simulink model "pendel_2016b"  (R2016b)
settings: Solver=ode45  StartTime=0.0  StopTime=30  RelTol=1e-5  AbsTol=1e-6
values from neighbouring files (symbols this model uses):
  fmax = 10    [pendel3.mat]
  g = 9.8    [pendel3.mat]    (also in stuff.m = 9.82)
  K = acker(A, B, P)    [stuff.m]
  l = 0.7    [pendel3.mat]    (also in stuff.m)
  L_1 = -10/(pi/6)    (= -19.098593171)    [stuff.m]
  L_2 = -8    [stuff.m]
  lam1 = -0.255    [pendel3.mat]
  m = 0.05    [pendel3.mat]
  M = 0.5    [pendel3.mat]    (also in stuff.m)
  ws = 1    [pendel3.mat]
  zs = 0.7    [pendel3.mat]
libraries: simulink x1
settings Model: ExtModeTrigMode=oneshot  ExtModeArmWhenConnect=off  Creator=bruze  LastModifiedBy=viktor
settings DataIOCC: SaveFormat=Array  SignalLoggingSaveFormat=ModelDataLogs
settings OptimizationCC: BlockReduction=off  BooleanDataType=off  ExpressionDepthLimit=2147483647  LifeSpan=inf
settings DebuggingCC: SaveWithParameterizedLinksMsg=none  UnderspecifiedInitializationDetection=Classic  MergeDetectMultiDrivingBlocksExec=none  SignalResolutionControl=TryResolveAllWithWarning  MultiTaskDSMMsg=warning  MultiTaskCondExecSysMsg=none  StateNameClashWarn=warning  SFUnexpectedBacktrackingDiag=warning  SFNoUnconditionalDefaultTransitionDiag=warning  SFExecutionAtInitializationDiag=none
settings HardwareCC: ProdBitPerPointer=32  ProdBitPerSizeT=32  ProdBitPerPtrDiffT=32  ProdLargestAtomicFloat=None  ProdIntDivRoundTo=Undefined  ProdEndianess=Unspecified  ProdWordSize=32  ProdHWDeviceType=32-bit Generic  TargetUnknown=on
settings ModelReferenceCC: PropagateSignalLabelsOutOfModel=off
settings GRTTargetCC: TargetLangStandard=C89/C90 (ANSI)  GeneratePreprocessorConditionals=Disable all  CombineOutputUpdateFcns=off  GRTInterface=on
settings ConfigComp: CovMetricSettings=dw  CovHtmlReporting=on  CovSaveCumulativeToWorkspaceVar=on  CovSaveSingleToWorkspaceVar=on  CovExternalEMLEnable=off  CovSFcnEnable=off

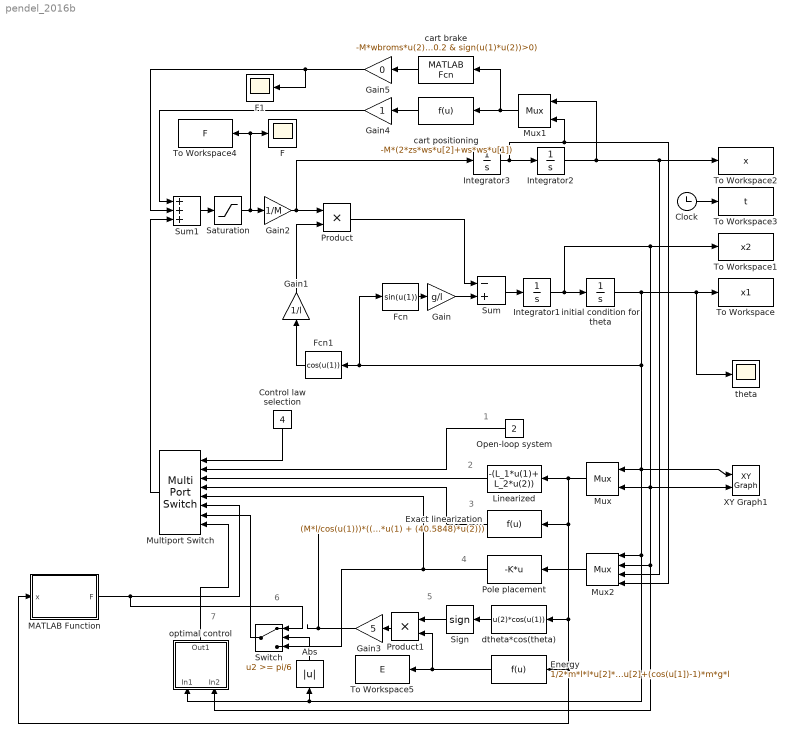
== system pendel_2016b ==
  note: 7
  note: 6
  note: 5
  note: 4
  note: 3
  note: 2
  note: 1
  " Linearized" : Fcn  Expr=-(L_1*u(1)+ L_2*u(2))
  Abs : Abs  SaturateOnIntegerOverflow=on
  Clock : Clock
  Control law selection : Constant  Value=4
  Energy : Fcn  Expr=1/2*m*l*l*u[2]*u[2]+(cos(u[1])-1)*m*g*l
  Exact linearization : Fcn  Expr=(M*l/cos(u(1)))*(((g/l)*sin(u(1))) + ((22.86)*u(1) + (40.5848)*u(2)))
  F : Scope
  F1 : Scope
  Fcn : Fcn  Expr=sin(u(1))
  Fcn1 : Fcn  Expr=cos(u(1))
  Gain : Gain  Gain=g/l  SaturateOnIntegerOverflow=on  OutDataTypeStr=Inherit: Same as input  ParamDataTypeStr=Inherit: Same as input
  Gain1 : Gain  Gain=1/l  SaturateOnIntegerOverflow=on  OutDataTypeStr=Inherit: Same as input  ParamDataTypeStr=Inherit: Same as input
  Gain2 : Gain  Gain=1/M  SaturateOnIntegerOverflow=on  OutDataTypeStr=Inherit: Same as input  ParamDataTypeStr=Inherit: Same as input
  Gain3 : Gain  Gain=5  SaturateOnIntegerOverflow=on  OutDataTypeStr=Inherit: Same as input  ParamDataTypeStr=Inherit: Same as input
  Gain4 : Gain  SaturateOnIntegerOverflow=on  OutDataTypeStr=Inherit: Same as input  ParamDataTypeStr=Inherit: Same as input
  Gain5 : Gain  Gain=0  SaturateOnIntegerOverflow=on  OutDataTypeStr=Inherit: Same as input  ParamDataTypeStr=Inherit: Same as input
  Integrator1 : Integrator
  Integrator2 : Integrator
  Integrator3 : Integrator
  MATLAB Function : MATLAB Function  TreatAsAtomicUnit=on
  Multiport Switch : MultiPortSwitch  Inputs=7  SaturateOnIntegerOverflow=on  InputSameDT=on
  Mux : Mux  Inputs=2
  Mux1 : Mux  Inputs=2
  Mux2 : Mux
  Open-loop system : Constant  Value=2
  Pole placement : MATLABFcn  MATLABFcn=-K*u  OutputDimensions=1
  Product : Product  SaturateOnIntegerOverflow=on  RndMeth=Zero  InputSameDT=on  OutDataTypeStr=Inherit: Same as first input
  Product1 : Product  SaturateOnIntegerOverflow=on  RndMeth=Zero  InputSameDT=on  OutDataTypeStr=Inherit: Same as first input
  Saturation : Saturate  UpperLimit=fmax  LowerLimit=-fmax
  Sign : Signum
  Sum : Sum  Inputs=-+  SaturateOnIntegerOverflow=on  InputSameDT=on  OutDataTypeStr=Inherit: Same as first input
  Sum1 : Sum  Inputs=+++  SaturateOnIntegerOverflow=on  InputSameDT=on  OutDataTypeStr=Inherit: Same as first input
  Switch : Switch  Threshold=pi/6  SaturateOnIntegerOverflow=on  InputSameDT=on
  To Workspace : ToWorkspace  VariableName=x1  SampleTime=-1
  To Workspace1 : ToWorkspace  VariableName=x2  SampleTime=-1
  To Workspace2 : ToWorkspace  VariableName=x  SampleTime=-1
  To Workspace3 : ToWorkspace  VariableName=t  SampleTime=-1
  To Workspace4 : ToWorkspace  VariableName=F  SampleTime=-1
  To Workspace5 : ToWorkspace  VariableName=E  SampleTime=-1
  XY Graph1 : simulink/Sinks/XY Graph  xmin=0  xmax=2*pi  ymin=-1  ymax=1  st=-1
  cart brake : MATLABFcn  MATLABFcn=-M*wbroms*u(2)*(abs(u(1))>0.2 & sign(u(1)*u(2))>0)  OutputDimensions=1
  cart positioning : Fcn  Expr=-M*(2*zs*ws*u[2]+ws*ws*u[1])
  dtheta*cos(theta) : Fcn  Expr=u(2)*cos(u(1))
  "initial condition for theta " : Integrator  InitialCondition=20*pi/180
  optimal control : Subsystem
  theta : Scope
  wires:
  Mux1/1 -> cart brake/1, cart positioning/1
  optimal control/1(Out1) -> Multiport Switch/8
  Abs/1 -> Switch/2
  Pole placement/1 -> Switch/3, Multiport Switch/5
  Gain3/1 -> ?
  Switch/1 -> Multiport Switch/7
  Mux2/1 -> Pole placement/1
  Gain5/1 -> F1/1, Sum1/2
  Multiport Switch/1 -> Sum1/3
  cart brake/1 -> Gain5/1
  Energy/1 -> To Workspace5/1, Product1/2
  Product1/1 -> Gain3/1
  Sign/1 -> Product1/1
  dtheta*cos(theta)/1 -> Sign/1
  Control law selection/1 -> Multiport Switch/1
  Open-loop system/1 -> Multiport Switch/2
  Mux/1 -> MATLAB Function/1(x), Energy/1, dtheta*cos(theta)/1, Exact linearization/1, " Linearized"/1
  " Linearized"/1 -> Multiport Switch/3
  Exact linearization/1 -> Multiport Switch/4
  Gain4/1 -> Sum1/1
  cart positioning/1 -> Gain4/1
  Sum1/1 -> Saturation/1
  Clock/1 -> To Workspace3/1
  Saturation/1 -> To Workspace4/1, F/1, Gain2/1
  Gain2/1 -> Product/1, Integrator3/1
  Product/1 -> Sum/1
  Gain1/1 -> Product/2
  Fcn1/1 -> Gain1/1
  Gain/1 -> Sum/2
  "initial condition for theta "/1 -> XY Graph1/1, optimal control/1(In1), Abs/1, Mux2/1, Mux/1, Fcn/1, Fcn1/1, To Workspace/1, theta/1
  Integrator1/1 -> To Workspace1/1, XY Graph1/2, Mux2/2, optimal control/2(In2), Mux/2, "initial condition for theta "/1
  Fcn/1 -> Gain/1
  Sum/1 -> Integrator1/1
  Integrator3/1 -> Integrator2/1, Mux1/2, Mux2/4
  Integrator2/1 -> Mux1/1, To Workspace2/1, Mux2/3
  MATLAB Function/1(F) -> Switch/1, Multiport Switch/6

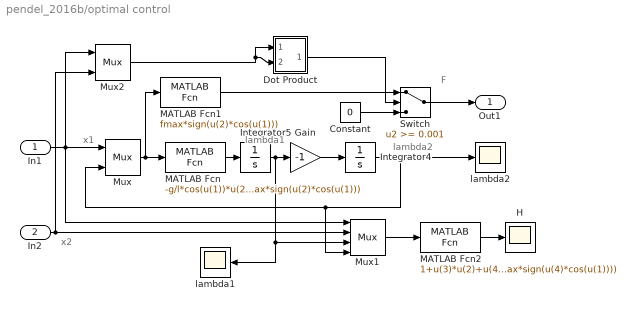
== system pendel_2016b/optimal control ==
  note: x2
  note: F
  note: x1
  note: lambda2
  note: lambda1
  In1 : Inport
  In2 : Inport  Port=2
  Constant : Constant  Value=0
  Dot Product : Subsystem  mask(Dot Product){}
      mask help:
      | Inner (dot) product.
      | y=sum(u1.*u2)
      mask init:
      | t=(0:.1:2*pi)';
      | x=cos(t);
      | y=sin(t);
      mask Help: Computes the inner (dot) product of the inputs: sum(u1.*u2).  The inputs are vectors of the same length. Output is a scalar.
      mask Display: plot(0,0,1,1,x*[0.025 0.07]+0.5,y*[0.025 0.07]+0.5)
  Gain : Gain  Gain=-1  SaturateOnIntegerOverflow=on  OutDataTypeStr=Inherit: Same as input  ParamDataTypeStr=Inherit: Same as input
  H : Scope
  Integrator4 : Integrator  InitialCondition=0.035
  Integrator5 : Integrator  InitialCondition=lam1
  MATLAB Fcn : MATLABFcn  MATLABFcn=-g/l*cos(u(1))*u(2)-1/(M*l)*sin(u(1))*u(2)*fmax*sign(u(2)*cos(u(1)))  OutputDimensions=1
  MATLAB Fcn1 : MATLABFcn  MATLABFcn=fmax*sign(u(2)*cos(u(1)))  OutputDimensions=1
  MATLAB Fcn2 : MATLABFcn  MATLABFcn=1+u(3)*u(2)+u(4)*(g/l*sin(u(1))-1/(M*l)*cos(u(1))*fmax*sign(u(4)*cos(u(1))))  OutputDimensions=1
  Mux : Mux  Inputs=2
  Mux1 : Mux
  Mux2 : Mux  Inputs=2
  Switch : Switch  Threshold=0.001  SaturateOnIntegerOverflow=on  InputSameDT=on
  lambda1 : Scope
  lambda2 : Scope
  Out1 : Outport  InitialOutput=0
  wires:
  Constant/1 -> Switch/3
  Gain/1 -> Integrator4/1
  MATLAB Fcn/1 -> Integrator5/1
  Switch/1 -> Out1/1
  Dot Product/1(out_1) -> Switch/2
  MATLAB Fcn1/1 -> Switch/1
  Mux2/1 -> Dot Product/2(in_2), Dot Product/1(in_1)
  In2/1 -> Mux2/2, Mux1/2
  Integrator4/1 -> lambda2/1, Mux1/4, Mux/2
  Integrator5/1 -> lambda1/1, Mux1/3, Gain/1
  MATLAB Fcn2/1 -> H/1
  Mux1/1 -> MATLAB Fcn2/1
  In1/1 -> Mux2/1, Mux1/1, Mux/1
  Mux/1 -> MATLAB Fcn1/1, MATLAB Fcn/1

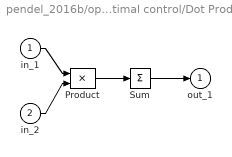
== system pendel_2016b/optimal control/Dot Product ==
  in_1 : Inport
  in_2 : Inport  Port=2
  Product : Product  SaturateOnIntegerOverflow=on  RndMeth=Zero  InputSameDT=on  OutDataTypeStr=Inherit: Same as first input
  Sum : Sum  Inputs=+  SaturateOnIntegerOverflow=on  InputSameDT=on  OutDataTypeStr=Inherit: Same as first input
  out_1 : Outport  InitialOutput=0
  wires:
  Sum/1 -> out_1/1
  Product/1 -> Sum/1
  in_1/1 -> Product/1
  in_2/1 -> Product/2

== matlab function pendel_2016b/MATLAB Function ==
  data: x input; F output
function F = fcn(x)
    l = 0.7;
    M = 0.5;
    m = 0.5;
    g = 9.82;

    alpha = 10;
    
    F = alpha/2 * ...
        (M/(m*l*x(2)*cos(x(1))) * ...
        ((m*x(2)^2*l^2/2) - ...
        (l*m*g*(1 - cos(x(1))))));
end
